simulink model "windTurbine_model"  (R2022b)
settings: Solver=VariableStepAuto  StartTime=0.0  StopTime=t_sample*n_sample  MaxStep=5  MinStep=1  RelTol=1e-3
values from neighbouring files (symbols this model uses):
  l1 = 56    [wind_turbine_parameters.m]
  t_sample = 10*60    (= 600)    [wind_turbine_parameters.m]
libraries: simulink x1, spsWindTurbineLib x1
settings Model: Creator=luan  LastModifiedBy=luan
settings SolverCC: ZeroCrossAlgorithm=Adaptive
settings DebuggingCC: IgnoredZcDiagnostic=none
settings ConfigComp: CovScope=ReferencedModels

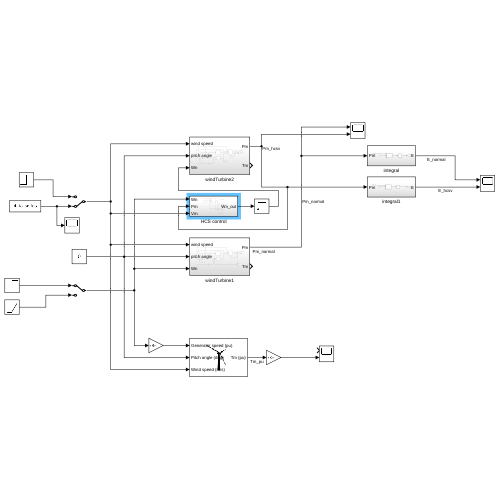
[thumbnail: Simulink's stored preview of the top-level diagram]
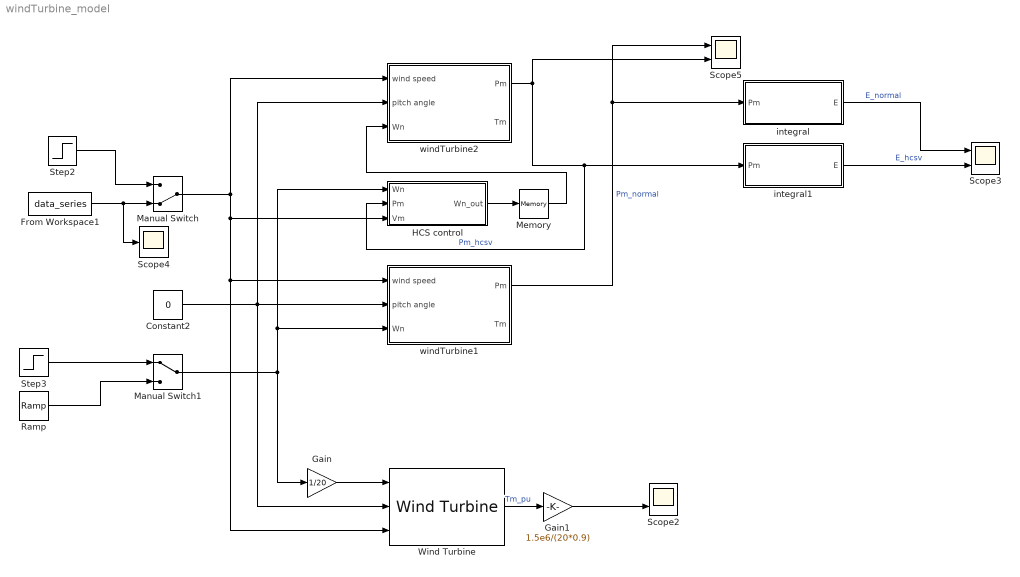
== system windTurbine_model ==
  Constant2 : Constant  Value=0
  From Workspace1 : FromWorkspace  VariableName=data_series  SampleTime=t_sample  OutputAfterFinalValue=Setting to zero
  Gain : Gain  Gain=1/20
  Gain1 : Gain  Gain=1.5e6/(20*0.9)
  HCS control : Subsystem
  Manual Switch : ManualSwitch  CurrentSetting=0
  Manual Switch1 : ManualSwitch
  Memory : Memory
  Ramp : simulink/Sources/Ramp  slope=0.000007  start=0  InitialOutput=0.0001
  Scope2 : Scope  NumInputPorts=2
  Scope3 : Scope  NumInputPorts=2
  Scope4 : Scope
  Scope5 : Scope  NumInputPorts=2
  Step2 : Step  Time=0  After=8  SampleTime=0
  Step3 : Step  Time=0  SampleTime=0
  Wind Turbine : spsWindTurbineLib/Wind Turbine  Pnom=1.5e6  Pelec_base=1.5e6/0.9  wind_base=20  P_wind_base=0.73  speed_nom=1.2  pitch_angle=0  c1_c6="[0.51763          116          0.4            5           21     0.006795]"  cp_nom=0.48  lambda_nom=8.1
  integral : Subsystem
  integral1 : Subsystem
  windTurbine1 : Subsystem
  windTurbine2 : Subsystem
  wires:
  Constant2/1 -> windTurbine2/2(pitch angle), Wind Turbine/2, windTurbine1/2(pitch angle)
  Gain/1 -> Wind Turbine/1
  Wind Turbine/1 -> Gain1/1  "Tm_pu"
  Gain1/1 -> Scope2/2
  windTurbine1/1(Pm) -> Scope5/1, integral/1(Pm)  "Pm_normal"
  windTurbine2/1(Pm) -> HCS control/2(Pm), integral1/1(Pm), Scope5/2  "Pm_hcsv"
  Step2/1 -> Manual Switch/1
  Manual Switch/1 -> Wind Turbine/3, windTurbine1/1(wind speed), HCS control/3(Vm), windTurbine2/1(wind speed)
  From Workspace1/1 -> Scope4/1, Manual Switch/2
  Step3/1 -> Manual Switch1/1
  Ramp/1 -> Manual Switch1/2
  Manual Switch1/1 -> HCS control/1(Wn), windTurbine1/3(Wn), Gain/1
  HCS control/1(Wn_out) -> Memory/1
  integral1/1(E) -> Scope3/2  "E_hcsv"
  Memory/1 -> windTurbine2/3(Wn)
  integral/1(E) -> Scope3/1  "E_normal"

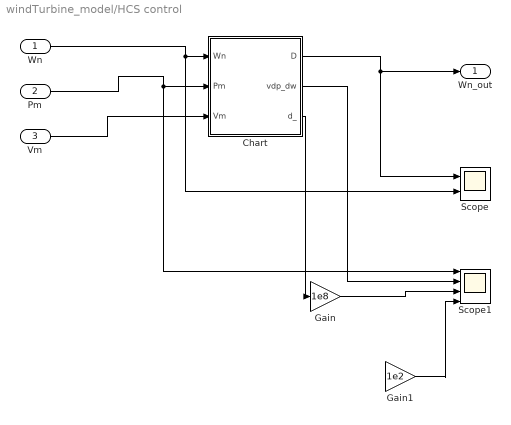
== system windTurbine_model/HCS control ==
  Wn : Inport
  Pm : Inport  Port=2
  Vm : Inport  Port=3
  Chart : Stateflow chart  TreatAsAtomicUnit=on
  Gain : Gain  Gain=1e8
  Gain1 : Gain  Gain=1e2
  Scope : Scope  NumInputPorts=2
  Scope1 : Scope  NumInputPorts=4
  Wn_out : Outport
  wires:
  Wn/1 -> Scope/2, Chart/1(Wn)
  Chart/1(D) -> Scope/1, Wn_out/1
  Vm/1 -> Chart/3(Vm)
  Chart/2(vdp_dw) -> Scope1/2
  Pm/1 -> Scope1/1, Chart/2(Pm)
  Gain/1 -> Scope1/3
  Chart/3(d_) -> Gain/1
  Gain1/1 -> Scope1/4
  ? -> Gain1/1

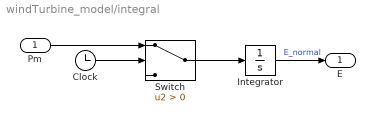
== system windTurbine_model/integral ==
  Pm : Inport
  Clock : Clock
  Integrator : Integrator
  Switch : Switch  Criteria=u2 > Threshold  SaturateOnIntegerOverflow=off  InputSameDT=off
  E : Outport
  wires:
  Switch/1 -> Integrator/1
  Clock/1 -> Switch/2
  Pm/1 -> Switch/1
  Integrator/1 -> E/1  "E_normal"

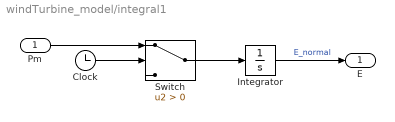
== system windTurbine_model/integral1 ==
  Pm : Inport
  Clock : Clock
  Integrator : Integrator
  Switch : Switch  Criteria=u2 > Threshold  SaturateOnIntegerOverflow=off  InputSameDT=off
  E : Outport
  wires:
  Integrator/1 -> E/1  "E_normal"
  Pm/1 -> Switch/1
  Clock/1 -> Switch/2
  Switch/1 -> Integrator/1

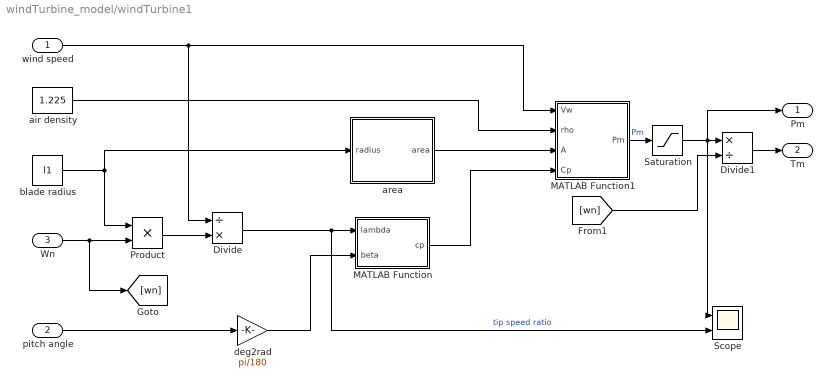
== system windTurbine_model/windTurbine1 ==
  wind speed : Inport
  pitch angle : Inport  Port=2
  Wn : Inport  Port=3
  Divide : Product  Inputs=/*
  Divide1 : Product  Inputs=*/
  MATLAB Function : MATLAB Function  TreatAsAtomicUnit=on
  MATLAB Function1 : MATLAB Function  TreatAsAtomicUnit=on
  Product : Product
  Saturation : Saturate  UpperLimit=inf  LowerLimit=0
  Scope : Scope  NumInputPorts=2
  air density : Constant  Value=1.225
  area : Subsystem
  blade radius : Constant  Value=l1
  deg2rad : Gain  Gain=pi/180
  Pm : Outport
  Tm : Outport  Port=2
  wires:
  MATLAB Function/1(cp) -> MATLAB Function1/4(Cp)
  Wn/1 -> [wn], Product/2
  Divide1/1 -> Tm/1
  [wn] -> Divide1/2
  MATLAB Function1/1(Pm) -> Saturation/1  "Pm"
  area/1(area) -> MATLAB Function1/3(A)
  air density/1 -> MATLAB Function1/2(rho)
  pitch angle/1 -> deg2rad/1
  Divide/1 -> Scope/2, MATLAB Function/1(lambda)  "tip speed ratio"
  wind speed/1 -> Divide/1, MATLAB Function1/1(Vw)
  Product/1 -> Divide/2
  blade radius/1 -> area/1(radius), Product/1
  deg2rad/1 -> MATLAB Function/2(beta)
  Saturation/1 -> Scope/1, Pm/1, Divide1/1

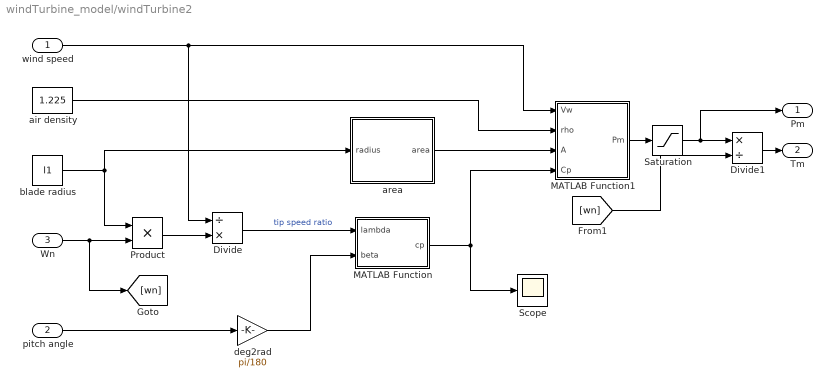
== system windTurbine_model/windTurbine2 ==
  wind speed : Inport
  pitch angle : Inport  Port=2
  Wn : Inport  Port=3
  Divide : Product  Inputs=/*
  Divide1 : Product  Inputs=*/
  MATLAB Function : MATLAB Function  TreatAsAtomicUnit=on
  MATLAB Function1 : MATLAB Function  TreatAsAtomicUnit=on
  Product : Product
  Saturation : Saturate  UpperLimit=inf  LowerLimit=0
  Scope : Scope
  air density : Constant  Value=1.225
  area : Subsystem
  blade radius : Constant  Value=l1
  deg2rad : Gain  Gain=pi/180
  Pm : Outport
  Tm : Outport  Port=2
  wires:
  deg2rad/1 -> MATLAB Function/2(beta)
  blade radius/1 -> Product/1, area/1(radius)
  Product/1 -> Divide/2
  wind speed/1 -> MATLAB Function1/1(Vw), Divide/1
  Divide/1 -> MATLAB Function/1(lambda)  "tip speed ratio"
  pitch angle/1 -> deg2rad/1
  air density/1 -> MATLAB Function1/2(rho)
  area/1(area) -> MATLAB Function1/3(A)
  [wn] -> Divide1/2
  Divide1/1 -> Tm/1
  Wn/1 -> Product/2, [wn]
  MATLAB Function/1(cp) -> Scope/1, MATLAB Function1/4(Cp)
  MATLAB Function1/1(Pm) -> Saturation/1
  Saturation/1 -> Pm/1, Divide1/1

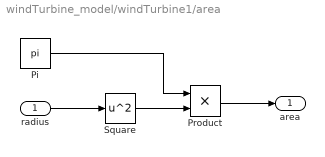
== system windTurbine_model/windTurbine1/area ==
  radius : Inport
  Pi : Constant  Value=pi  OutDataTypeStr=Inherit: Inherit via back propagation
  Product : Product
  Square : Math  Operator=square
  area : Outport
  wires:
  Product/1 -> area/1
  Pi/1 -> Product/1
  Square/1 -> Product/2
  radius/1 -> Square/1

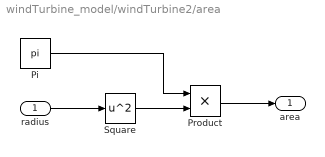
== system windTurbine_model/windTurbine2/area ==
  radius : Inport
  Pi : Constant  Value=pi  OutDataTypeStr=Inherit: Inherit via back propagation
  Product : Product
  Square : Math  Operator=square
  area : Outport
  wires:
  radius/1 -> Square/1
  Square/1 -> Product/2
  Pi/1 -> Product/1
  Product/1 -> area/1

== matlab function windTurbine_model/windTurbine1/MATLAB Function ==
  data: lambda input; cp output; beta input
function cp = fcn(lambda, beta)

model = 'kumar_model';

if(strcmp(model, 'kumar_model'))
    %disp(model)
    k = load('coefficients.mat');
    lambda_i =  1/(1/(lambda + 0.08*beta) - 0.035/(1+beta^3));
    cp = k.k1 *(k.k2/lambda_i - k.k3*beta - k.k4*beta^(k.k5) -k.k6)*exp(-k.k7/lambda_i);
end
if(strcmp(model, 'matlab_model'))
    %disp(model)
    k = load('coefficients_matlab_model.mat');
    lambda_i =  1/(1/(lambda + 0.08*beta) - 0.035/(1+beta*beta*beta));
    cp = k.k1*( k.k2/lambda_i - k.k3*beta - k.k4 )*exp( -k.k5/lambda_i ) + k.k6*lambda;
end

== matlab function windTurbine_model/windTurbine1/MATLAB Function1 ==
  data: Vw input; Pm output; rho input; A input; Cp input
function Pm = fcn(Vw, rho, A, Cp)

Pm = 0.5* Cp* rho* A* Vw^3;

== matlab function windTurbine_model/windTurbine2/MATLAB Function ==
  data: lambda input; cp output; beta input
function cp = fcn(lambda, beta)

model = 'kumar_model';

if(strcmp(model, 'kumar_model'))
    %disp(model)
    k = load('coefficients.mat');
    lambda_i =  1/(1/(lambda + 0.08*beta) - 0.035/(1+beta^3));
    cp = k.k1 *(k.k2/lambda_i - k.k3*beta - k.k4*beta^(k.k5) -k.k6)*exp(-k.k7/lambda_i);
end
if(strcmp(model, 'matlab_model'))
    %disp(model)
    k = load('coefficients_matlab_model.mat');
    lambda_i =  1/(1/(lambda + 0.08*beta) - 0.035/(1+beta*beta*beta));
    cp = k.k1*( k.k2/lambda_i - k.k3*beta - k.k4 )*exp( -k.k5/lambda_i ) + k.k6*lambda;
end

== matlab function windTurbine_model/windTurbine2/MATLAB Function1 ==
  data: Vw input; Pm output; rho input; A input; Cp input
function Pm = fcn(Vw, rho, A, Cp)

Pm = 0.5* Cp* rho* A* Vw^3;

== stateflow chart windTurbine_model/HCS control/Chart ==
  state stationary
    entry:
    D = Wn;
  state measure
    entry:
    dp = Pm - pt_1;
    dw = D-wn_1;
    pt_1 = Pm;
    wn_1 = D;
    vdp_dw =  Vm*dp/dw;
  state decrease
    entry:
  state decrease_a_lot
    entry:
    d_ = - d_lot;
  state init_
    entry:
    D = Wn;
    pt_1 = 0;
    wn_1 = 0;
    vdp_dw_1 = 0;
  state decrease_a_bit
    entry:
    d_ = - d_bit;
  state perturb_
    entry:
    D = D + d_;
    vdp_dw_1 = vdp_dw;
  state increase_a_bit
    entry:
    d_ = d_bit;
  state increase
    entry:
  state increase_a_lot
    entry:
    d_ = d_lot;
  measure -> stationary [order 3] : [dp==0]
  stationary -> measure : [after(delay,sec)]
  (junction 73) -> (junction 74)
  (junction 74) -> measure
  (junction 77) -> (junction 73)
  (default) -> init_
  decrease_a_lot -> (junction 66)
  measure -> decrease [order 2] : [dp < 0]
  decrease -> decrease_a_lot [order 2] : [Pm < vdp_dw_1]
  (junction 66) -> perturb_
  init_ -> measure
  decrease -> decrease_a_bit [order 1] : [Pm > vdp_dw_1]
  measure -> increase [order 1] : [dp > 0]
  decrease_a_bit -> (junction 70)
  (junction 70) -> perturb_
  perturb_ -> (junction 77) : [after(delay,sec)]
  (junction 63) -> perturb_
  (junction 60) -> perturb_
  increase_a_bit -> (junction 63)
  increase -> increase_a_bit [order 1] : [Pm > vdp_dw_1]
  increase -> (junction 45) [order 2] : [Pm < vdp_dw_1]
  (junction 45) -> increase_a_lot
  increase_a_lot -> (junction 60)
  data: Wn input; Pm input; D output; delay constant double =60; d_bit constant double =0.005; pt_1 local; wn_1 local; d_lot local double =0.15; Vm input; dw local; vdp_dw output; d_ output; vdp_dw_1 local; dp local
